simulink model "RT_ueb3_2block"  (R2013a)
settings: Solver=ode45  StartTime=0.0  StopTime=10.0  RelTol=1e-3
values from neighbouring files (symbols this model uses):
  k = 1    [RT_Klausur_SS2014.m]    (also in RT_ctrl_analyse_proc.m = 5; RT_dennis_draussen.m = 50; RT_klausurvorb.m = 0.2; RT_lab_paramLead.m)
settings Model: Creator=mainster  LastModifiedBy=mainster

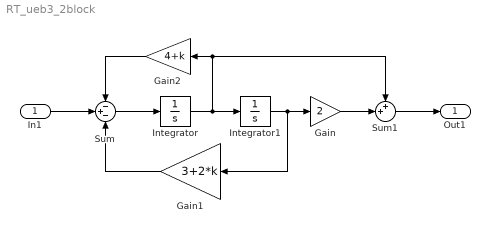
== system RT_ueb3_2block ==
  In1 : Inport
  Gain : Gain  Gain=2
  Gain1 : Gain  Gain=3+2*k
  Gain2 : Gain  Gain=4+k
  Integrator : Integrator
  Integrator1 : Integrator
  Sum : Sum  Inputs=-+-
  Sum1 : Sum  Inputs=++|
  Out1 : Outport
  wires:
  Gain2/1 -> Sum/1
  Gain1/1 -> Sum/3
  Sum/1 -> Integrator/1
  Integrator/1 -> Sum1/1, Gain2/1, Integrator1/1
  Integrator1/1 -> Gain1/1, Gain/1
  Gain/1 -> Sum1/2
  In1/1 -> Sum/2
  Sum1/1 -> Out1/1
